simulink model "tasks100Hz"  (R2014a)
settings: Solver=FixedStepDiscrete  StartTime=0.0  StopTime=simTime  FixedStep=filterDT  RelTol=1e-3
values from neighbouring files (symbols this model uses):
  earthAccelDenHP = p    [setup.m]
  earthAccelNumHP = p    [setup.m]
  eepromConfig = p    [setup.m]
  filterDT = 1 / 100    (= 0.01)    [setup.m]
undefined symbols (not defined in the file or in its folder): DiscIntNeverNeededParam
libraries: simulink x7, aerolibutil x4, aerolibtransform2 x1
settings Model: Creator=John Ihlein  LastModifiedBy=John Ihlein
settings DataIOCC: SaveFormat=Structure  SaveOutput=off  SaveTime=off
settings OptimizationCC: InlineParams=on  DefaultUnderspecifiedDataType=single  InlineInvariantSignals=on  PassReuseOutputArgsAs=Individual arguments  StateBitsets=on  DataBitsets=on  ZeroExternalMemoryAtStartup=off  ZeroInternalMemoryAtStartup=off  EfficientFloat2IntCast=on  OptimizeModelRefInitCode=on  LifeSpan=1
settings DebuggingCC: ParameterPrecisionLossMsg=none  UniqueDataStoreMsg=error  AssertControl=DisableAll
settings HardwareCC: ProdLargestAtomicInteger=Integer  ProdLargestAtomicFloat=Float  ProdIntDivRoundTo=Zero  ProdEndianess=LittleEndian  ProdHWDeviceType=STMicroelectronics->STM32F4xx 32-bit Cortex-M4
settings RTWCC: SystemTargetFile=ert.tlc  GenCodeOnly=on  TemplateMakefile=ert_default_tmf  Description=Embedded Coder  ProcessScript=ert_make_rtw_hook
settings CodeAppCC: IgnoreCustomStorageClasses=off  IgnoreTestpoints=on
settings ERTTargetCC: ParMdlRefBuildCompliant=on  CompOptLevelCompliant=on  ConcurrentExecutionCompliant=on  IncludeMdlTerminateFcn=off  ERTFirstTimeCompliant=on  SupportNonFinite=off  ParenthesesLevel=Maximum  ModelStepFunctionPrototypeControlCompliant=on  CPPClassGenCompliant=on  InlinedParameterPlacement=Hierarchical  ERTCustomFileTemplate=example_file_process.tlc  ERTFilePackagingFormat=Compact

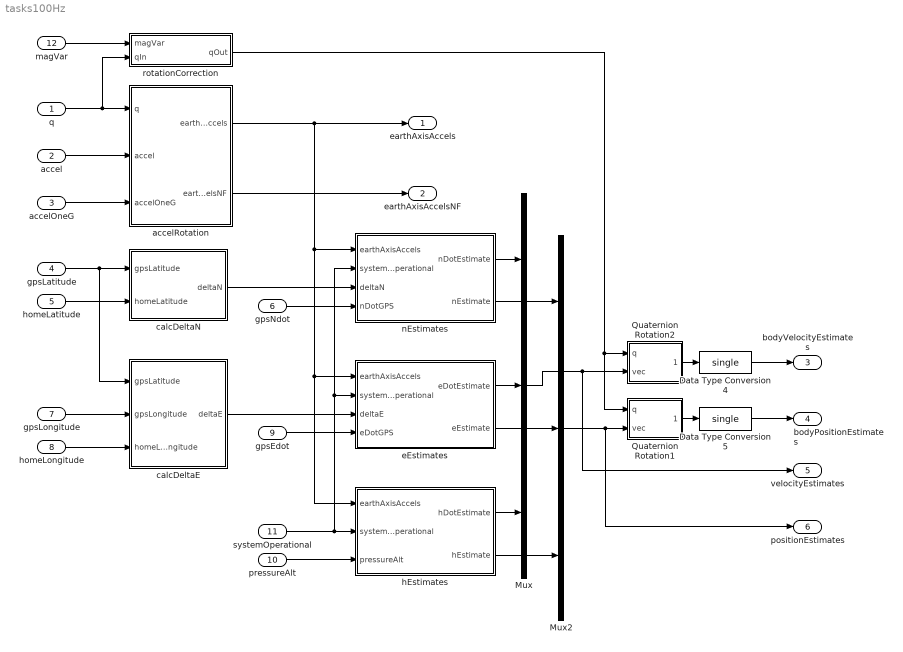
== system tasks100Hz ==
  q : Inport  OutDataTypeStr=single  PortDimensions=4  SampleTime=filterDT
  accel : Inport  Port=2  OutDataTypeStr=single  PortDimensions=3  SampleTime=filterDT
  accelOneG : Inport  Port=3  OutDataTypeStr=single  PortDimensions=1  SampleTime=filterDT
  gpsLatitude : Inport  Port=4  OutDataTypeStr=int32  PortDimensions=1  SampleTime=filterDT
  homeLatitude : Inport  Port=5  OutDataTypeStr=int32  PortDimensions=1  SampleTime=filterDT
  gpsNdot : Inport  Port=6  OutDataTypeStr=int32  PortDimensions=1  SampleTime=filterDT
  gpsLongitude : Inport  Port=7  OutDataTypeStr=int32  PortDimensions=1  SampleTime=filterDT
  homeLongitude : Inport  Port=8  OutDataTypeStr=int32  PortDimensions=1  SampleTime=filterDT
  gpsEdot : Inport  Port=9  OutDataTypeStr=int32  PortDimensions=1  SampleTime=filterDT
  pressureAlt : Inport  Port=10  OutDataTypeStr=single  PortDimensions=1  SampleTime=filterDT
  systemOperational : Inport  Port=11  OutDataTypeStr=uint8  PortDimensions=1  SampleTime=filterDT
  magVar : Inport  Port=12  OutDataTypeStr=single  PortDimensions=1  SampleTime=filterDT
  Data Type Conversion4 : DataTypeConversion  OutDataTypeStr=single
  Data Type Conversion5 : DataTypeConversion  OutDataTypeStr=single
  Mux : Mux  Inputs=3
  Mux2 : Mux  Inputs=3
  Quaternion Rotation1 : Subsystem
  Quaternion Rotation2 : Subsystem
  accelRotation : Subsystem  TreatAsAtomicUnit=on
  calcDeltaE : Subsystem  TreatAsAtomicUnit=on
  calcDeltaN : Subsystem  TreatAsAtomicUnit=on
  eEstimates : Subsystem  TreatAsAtomicUnit=on
  hEstimates : Subsystem  TreatAsAtomicUnit=on
  nEstimates : Subsystem  TreatAsAtomicUnit=on
  rotationCorrection : Subsystem  TreatAsAtomicUnit=on
  earthAxisAccels : Outport  OutDataTypeStr=single  PortDimensions=3  SampleTime=filterDT
  earthAxisAccelsNF : Outport  Port=2  OutDataTypeStr=single  PortDimensions=3  SampleTime=filterDT
  bodyVelocityEstimates : Outport  Port=3  OutDataTypeStr=single  PortDimensions=3  SampleTime=filterDT
  bodyPositionEstimates : Outport  Port=4  OutDataTypeStr=single  PortDimensions=3  SampleTime=filterDT
  velocityEstimates : Outport  Port=5  OutDataTypeStr=single  PortDimensions=3  SampleTime=filterDT
  positionEstimates : Outport  Port=6  OutDataTypeStr=single  PortDimensions=3  SampleTime=filterDT
  wires:
  systemOperational/1 -> nEstimates/2(systemOperational), eEstimates/2(systemOperational), hEstimates/2(systemOperational)
  pressureAlt/1 -> hEstimates/3(pressureAlt)
  hEstimates/1(hDotEstimate) -> Mux/3
  gpsNdot/1 -> nEstimates/4(nDotGPS)
  gpsEdot/1 -> eEstimates/4(eDotGPS)
  nEstimates/1(nDotEstimate) -> Mux/1
  nEstimates/2(nEstimate) -> Mux2/1
  eEstimates/1(eDotEstimate) -> Mux/2
  eEstimates/2(eEstimate) -> Mux2/2
  Quaternion Rotation2/1(vec_rot) -> Data Type Conversion4/1
  Quaternion Rotation1/1(vec_rot) -> Data Type Conversion5/1
  Data Type Conversion4/1 -> bodyVelocityEstimates/1
  Data Type Conversion5/1 -> bodyPositionEstimates/1
  hEstimates/2(hEstimate) -> Mux2/3
  Mux2/1 -> positionEstimates/1, Quaternion Rotation1/2(vec)
  accelOneG/1 -> accelRotation/3(accelOneG)
  homeLatitude/1 -> calcDeltaN/2(homeLatitude)
  calcDeltaN/1(deltaN) -> nEstimates/3(deltaN)
  gpsLongitude/1 -> calcDeltaE/2(gpsLongitude)
  homeLongitude/1 -> calcDeltaE/3(homeLongitude)
  calcDeltaE/1(deltaE) -> eEstimates/3(deltaE)
  gpsLatitude/1 -> calcDeltaN/1(gpsLatitude), calcDeltaE/1(gpsLatitude)
  q/1 -> rotationCorrection/2(qIn), accelRotation/1(q)
  accelRotation/2(earthAxisAccelsNF) -> earthAxisAccelsNF/1
  accelRotation/1(earthAxisAccels) -> eEstimates/1(earthAxisAccels), hEstimates/1(earthAxisAccels), nEstimates/1(earthAxisAccels), earthAxisAccels/1
  accel/1 -> accelRotation/2(accel)
  Mux/1 -> velocityEstimates/1, Quaternion Rotation2/2(vec)
  magVar/1 -> rotationCorrection/1(magVar)
  rotationCorrection/1(qOut) -> Quaternion Rotation2/1(q), Quaternion Rotation1/1(q)

== system tasks100Hz/Quaternion Rotation1 ==
  q : Inport
  vec : Inport  Port=2
  Mux1 : Mux  Inputs=3
  Quaternion Normalize : aerolibutil/Quaternion Normalize
  singleV1 : Subsystem
  singleV2 : Subsystem
  singleV3 : Subsystem
  vec_rot : Outport
  wires:
  q/1 -> Quaternion Normalize/1
  singleV1/1(V1) -> Mux1/1
  vec/1 -> singleV1/2(vec), singleV3/2(vec), singleV2/2(vec)
  Quaternion Normalize/1 -> singleV1/1(q), singleV3/1(q), singleV2/1(q)
  Mux1/1 -> vec_rot/1
  singleV3/1(V3) -> Mux1/3
  singleV2/1(V2) -> Mux1/2

== system tasks100Hz/Quaternion Rotation2 ==
  q : Inport
  vec : Inport  Port=2
  Mux1 : Mux  Inputs=3
  Quaternion Normalize : aerolibutil/Quaternion Normalize
  singleV1 : Subsystem
  singleV2 : Subsystem
  singleV3 : Subsystem
  vec_rot : Outport
  wires:
  singleV2/1(V2) -> Mux1/2
  singleV3/1(V3) -> Mux1/3
  Mux1/1 -> vec_rot/1
  Quaternion Normalize/1 -> singleV2/1(q), singleV3/1(q), singleV1/1(q)
  vec/1 -> singleV2/2(vec), singleV3/2(vec), singleV1/2(vec)
  singleV1/1(V1) -> Mux1/1
  q/1 -> Quaternion Normalize/1

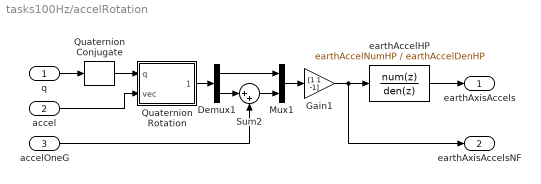
== system tasks100Hz/accelRotation ==
  q : Inport
  accel : Inport  Port=2
  accelOneG : Inport  Port=3
  Demux1 : Demux  Outputs=[2 1]
  Gain1 : Gain  Gain=[1 1 -1]
  Mux1 : Mux  Inputs=[2 1]
  Quaternion Conjugate : aerolibutil/Quaternion Conjugate
  Quaternion Rotation : Subsystem
  Sum2 : Sum  Inputs=|++
  earthAccelHP : DiscreteTransferFcn  Numerator=earthAccelNumHP  Denominator=earthAccelDenHP
  earthAxisAccels : Outport
  earthAxisAccelsNF : Outport  Port=2
  wires:
  Gain1/1 -> earthAxisAccelsNF/1, earthAccelHP/1
  accelOneG/1 -> Sum2/2
  Demux1/1 -> Mux1/1
  Sum2/1 -> Mux1/2
  Demux1/2 -> Sum2/1
  Quaternion Conjugate/1 -> Quaternion Rotation/1(q)
  accel/1 -> Quaternion Rotation/2(vec)
  q/1 -> Quaternion Conjugate/1
  Quaternion Rotation/1(vec_rot) -> Demux1/1
  Mux1/1 -> Gain1/1
  earthAccelHP/1 -> earthAxisAccels/1

== system tasks100Hz/calcDeltaE ==
  gpsLatitude : Inport
  gpsLongitude : Inport  Port=2
  homeLongitude : Inport  Port=3
  Data Type Conversion2 : DataTypeConversion  OutDataTypeStr=single
  Data Type Conversion3 : DataTypeConversion  OutDataTypeStr=single
  Gain1 : Gain  Gain=pi / 180 * 1e-7
  Gain2 : Gain  Gain=0.01111949
  Product : Product
  Sum2 : Sum  Inputs=|+-
  Trigonometric Function : Trigonometry  Operator=cos
  stdRadianLimit : Subsystem
  deltaE : Outport
  wires:
  stdRadianLimit/1(stdDegrees) -> Gain2/1
  gpsLatitude/1 -> Data Type Conversion2/1
  Data Type Conversion3/1 -> stdRadianLimit/1(degrees)
  Product/1 -> deltaE/1
  Sum2/1 -> Data Type Conversion3/1
  homeLongitude/1 -> Sum2/2
  Gain2/1 -> Product/2
  Trigonometric Function/1 -> Product/1
  Gain1/1 -> Trigonometric Function/1
  Data Type Conversion2/1 -> Gain1/1
  gpsLongitude/1 -> Sum2/1

== system tasks100Hz/calcDeltaN ==
  gpsLatitude : Inport
  homeLatitude : Inport  Port=2
  Data Type Conversion1 : DataTypeConversion  OutDataTypeStr=single
  Gain : Gain  Gain=0.01111949
  Sum1 : Sum  Inputs=|+-
  deltaN : Outport
  wires:
  Sum1/1 -> Data Type Conversion1/1
  homeLatitude/1 -> Sum1/2
  Data Type Conversion1/1 -> Gain/1
  gpsLatitude/1 -> Sum1/1
  Gain/1 -> deltaN/1

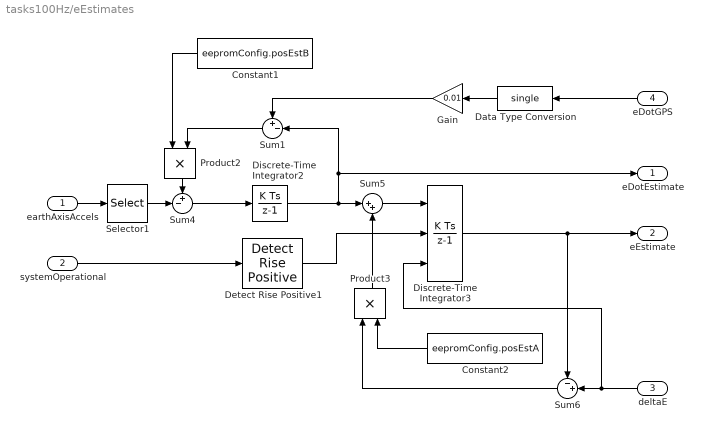
== system tasks100Hz/eEstimates ==
  earthAxisAccels : Inport
  systemOperational : Inport  Port=2
  deltaE : Inport  Port=3
  eDotGPS : Inport  Port=4  OutDataTypeStr=int32
  Constant1 : Constant  Value=eepromConfig.posEstB  SampleTime=filterDT
  Constant2 : Constant  Value=eepromConfig.posEstA  SampleTime=filterDT
  Data Type Conversion : DataTypeConversion  OutDataTypeStr=single
  Detect Rise Positive1 : simulink/Logic and Bit Operations/Detect Rise Positive  vinit=0  InputProcessing=Inherited  OutDataTypeStr=boolean
  Discrete-Time Integrator2 : DiscreteIntegrator  SampleTime=filterDT  ICPrevOutput=DiscIntNeverNeededParam  ICPrevScaledInput=DiscIntNeverNeededParam
  Discrete-Time Integrator3 : DiscreteIntegrator  ExternalReset=rising  InitialConditionSource=external  SampleTime=filterDT  ICPrevOutput=DiscIntNeverNeededParam  ICPrevScaledInput=DiscIntNeverNeededParam
  Gain : Gain  Gain=0.01
  Product2 : Product
  Product3 : Product
  Selector1 : Selector  IndexMode=Zero-based  InputPortWidth=3
  Sum1 : Sum  Inputs=+-|
  Sum4 : Sum  Inputs=+-|
  Sum5 : Sum  Inputs=|++
  Sum6 : Sum  Inputs=-+|
  eDotEstimate : Outport
  eEstimate : Outport  Port=2
  wires:
  Data Type Conversion/1 -> Gain/1
  Gain/1 -> Sum1/1
  eDotGPS/1 -> Data Type Conversion/1
  Sum1/1 -> Product2/2
  Constant1/1 -> Product2/1
  Product2/1 -> Sum4/1
  Selector1/1 -> Sum4/2
  Sum4/1 -> Discrete-Time Integrator2/1
  Product3/1 -> Sum5/2
  Detect Rise Positive1/1 -> Discrete-Time Integrator3/2
  Constant2/1 -> Product3/2
  Discrete-Time Integrator3/1 -> eEstimate/1, Sum6/1
  Sum6/1 -> Product3/1
  Discrete-Time Integrator2/1 -> eDotEstimate/1, Sum1/2, Sum5/1
  Sum5/1 -> Discrete-Time Integrator3/1
  earthAxisAccels/1 -> Selector1/1
  deltaE/1 -> Discrete-Time Integrator3/3, Sum6/2
  systemOperational/1 -> Detect Rise Positive1/1

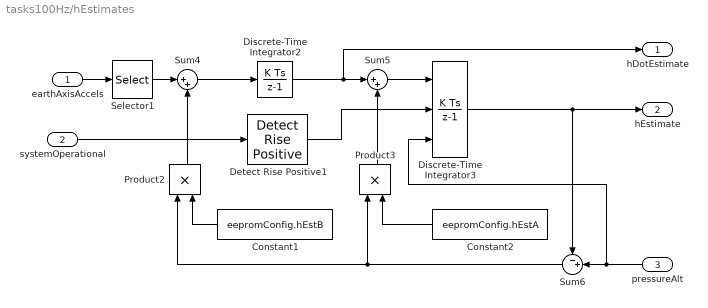
== system tasks100Hz/hEstimates ==
  earthAxisAccels : Inport
  systemOperational : Inport  Port=2
  pressureAlt : Inport  Port=3
  Constant1 : Constant  Value=eepromConfig.hEstB  SampleTime=filterDT
  Constant2 : Constant  Value=eepromConfig.hEstA  SampleTime=filterDT
  Detect Rise Positive1 : simulink/Logic and Bit Operations/Detect Rise Positive  vinit=0  InputProcessing=Inherited  OutDataTypeStr=boolean
  Discrete-Time Integrator2 : DiscreteIntegrator  SampleTime=filterDT  ICPrevOutput=DiscIntNeverNeededParam  ICPrevScaledInput=DiscIntNeverNeededParam
  Discrete-Time Integrator3 : DiscreteIntegrator  ExternalReset=rising  InitialConditionSource=external  SampleTime=filterDT  ICPrevOutput=DiscIntNeverNeededParam  ICPrevScaledInput=DiscIntNeverNeededParam
  Product2 : Product
  Product3 : Product
  Selector1 : Selector  IndexMode=Zero-based  InputPortWidth=3  Indices=2
  Sum4 : Sum  Inputs=|++
  Sum5 : Sum  Inputs=|++
  Sum6 : Sum  Inputs=-+|
  hDotEstimate : Outport
  hEstimate : Outport  Port=2
  wires:
  systemOperational/1 -> Detect Rise Positive1/1
  pressureAlt/1 -> Sum6/2, Discrete-Time Integrator3/3
  earthAxisAccels/1 -> Selector1/1
  Sum5/1 -> Discrete-Time Integrator3/1
  Discrete-Time Integrator2/1 -> Sum5/1, hDotEstimate/1
  Sum6/1 -> Product3/1, Product2/1
  Discrete-Time Integrator3/1 -> Sum6/1, hEstimate/1
  Constant2/1 -> Product3/2
  Selector1/1 -> Sum4/1
  Detect Rise Positive1/1 -> Discrete-Time Integrator3/2
  Product3/1 -> Sum5/2
  Sum4/1 -> Discrete-Time Integrator2/1
  Constant1/1 -> Product2/2
  Product2/1 -> Sum4/2

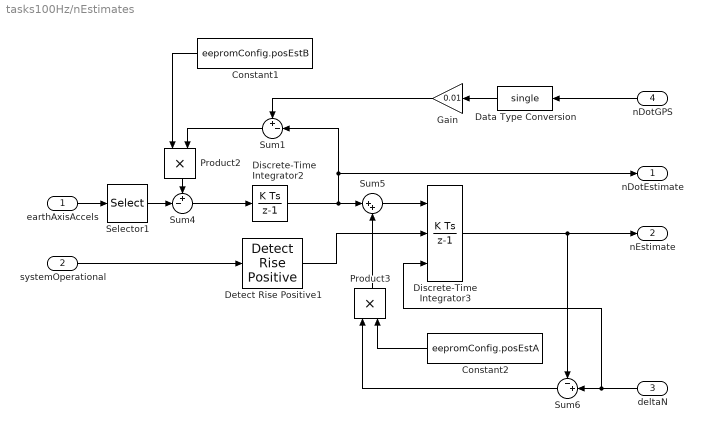
== system tasks100Hz/nEstimates ==
  earthAxisAccels : Inport
  systemOperational : Inport  Port=2
  deltaN : Inport  Port=3
  nDotGPS : Inport  Port=4  OutDataTypeStr=int32
  Constant1 : Constant  Value=eepromConfig.posEstB  SampleTime=filterDT
  Constant2 : Constant  Value=eepromConfig.posEstA  SampleTime=filterDT
  Data Type Conversion : DataTypeConversion  OutDataTypeStr=single
  Detect Rise Positive1 : simulink/Logic and Bit Operations/Detect Rise Positive  vinit=0  InputProcessing=Inherited  OutDataTypeStr=boolean
  Discrete-Time Integrator2 : DiscreteIntegrator  SampleTime=filterDT  ICPrevOutput=DiscIntNeverNeededParam  ICPrevScaledInput=DiscIntNeverNeededParam
  Discrete-Time Integrator3 : DiscreteIntegrator  ExternalReset=rising  InitialConditionSource=external  SampleTime=filterDT  ICPrevOutput=DiscIntNeverNeededParam  ICPrevScaledInput=DiscIntNeverNeededParam
  Gain : Gain  Gain=0.01
  Product2 : Product
  Product3 : Product
  Selector1 : Selector  IndexMode=Zero-based  InputPortWidth=3  Indices=0
  Sum1 : Sum  Inputs=+-|
  Sum4 : Sum  Inputs=+-|
  Sum5 : Sum  Inputs=|++
  Sum6 : Sum  Inputs=-+|
  nDotEstimate : Outport
  nEstimate : Outport  Port=2
  wires:
  systemOperational/1 -> Detect Rise Positive1/1
  deltaN/1 -> Sum6/2, Discrete-Time Integrator3/3
  earthAxisAccels/1 -> Selector1/1
  Sum5/1 -> Discrete-Time Integrator3/1
  Discrete-Time Integrator2/1 -> Sum5/1, Sum1/2, nDotEstimate/1
  Sum6/1 -> Product3/1
  Discrete-Time Integrator3/1 -> Sum6/1, nEstimate/1
  Constant2/1 -> Product3/2
  Detect Rise Positive1/1 -> Discrete-Time Integrator3/2
  Product3/1 -> Sum5/2
  Sum4/1 -> Discrete-Time Integrator2/1
  Selector1/1 -> Sum4/2
  Product2/1 -> Sum4/1
  Constant1/1 -> Product2/1
  Sum1/1 -> Product2/2
  nDotGPS/1 -> Data Type Conversion/1
  Gain/1 -> Sum1/1
  Data Type Conversion/1 -> Gain/1

== system tasks100Hz/rotationCorrection ==
  magVar : Inport
  qIn : Inport  Port=2
  Demux : Demux  Outputs=[1 2]
  Gain3 : Gain  Gain=[1 0 0]
  Mux : Mux  Inputs=[1 2]
  Quaternions to Rotation Angles : aerolibtransform2/Quaternions to Rotation Angles  rotationOrder=ZYX
  Rotation Angles to Quaternions Rotation Order: ZYX : Subsystem
  Sum : Sum  Inputs=++|
  stdRadianLimit : Subsystem
  qOut : Outport
  wires:
  Mux/1 -> Rotation Angles to Quaternions Rotation Order: ZYX/1("R1, R2, R3")
  Gain3/1 -> Demux/1
  stdRadianLimit/1(stdRadians) -> Mux/1
  Demux/1 -> Sum/2
  Demux/2 -> Mux/2
  magVar/1 -> Sum/1
  Sum/1 -> stdRadianLimit/1(radians)
  qIn/1 -> Quaternions to Rotation Angles/1
  Quaternions to Rotation Angles/1 -> Gain3/1
  Rotation Angles to Quaternions Rotation Order: ZYX/1(q) -> qOut/1

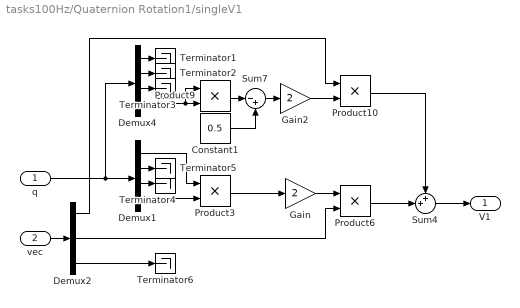
== system tasks100Hz/Quaternion Rotation1/singleV1 ==
  q : Inport
  vec : Inport  Port=2
  Constant1 : Constant  Value=0.5  OutDataTypeStr=single
  Demux1 : Demux
  Demux2 : Demux  Outputs=3
  Demux4 : Demux
  Gain : Gain  Gain=2
  Gain2 : Gain  Gain=2
  Product{3,6,9..10} (4 alike) : Product  RndMeth=Zero
  Sum4 : Sum  Inputs=++|
  Sum7 : Sum  Inputs=|-+
  Terminator{1..6} (6 alike) : Terminator
  V1 : Outport
  wires:
  Product6/1 -> Sum4/2
  Sum4/1 -> V1/1
  q/1 -> Demux4/1, Demux1/1
  vec/1 -> Demux2/1
  Demux1/4 -> Product3/2
  Demux1/1 -> Product3/1
  Product3/1 -> Gain/1
  Product10/1 -> Sum4/1
  Demux4/2 -> Terminator2/1
  Gain/1 -> Product6/1
  Gain2/1 -> Product10/2
  Demux2/2 -> Product6/2
  Demux2/1 -> Product10/1
  Sum7/1 -> Gain2/1
  Demux4/1 -> Terminator1/1
  Demux4/3 -> Terminator3/1
  Demux4/4 -> Product9/1, Product9/2
  Product9/1 -> Sum7/1
  Constant1/1 -> Sum7/2
  Demux1/3 -> Terminator4/1
  Demux1/2 -> Terminator5/1
  Demux2/3 -> Terminator6/1

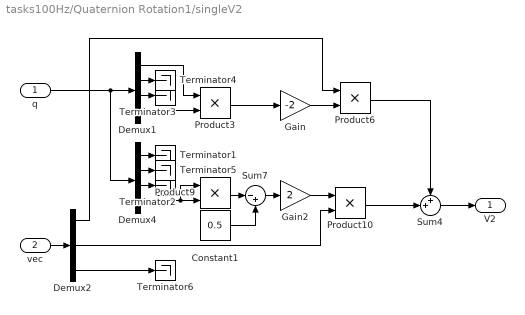
== system tasks100Hz/Quaternion Rotation1/singleV2 ==
  q : Inport
  vec : Inport  Port=2
  Constant1 : Constant  Value=0.5  OutDataTypeStr=single
  Demux1 : Demux
  Demux2 : Demux  Outputs=3
  Demux4 : Demux
  Gain : Gain  Gain=-2
  Gain2 : Gain  Gain=2
  Product{3,6,9..10} (4 alike) : Product  RndMeth=Zero
  Sum4 : Sum  Inputs=++|
  Sum7 : Sum  Inputs=|-+
  Terminator{1..6} (6 alike) : Terminator
  V2 : Outport
  wires:
  Demux1/1 -> Product3/1
  Demux1/4 -> Product3/2
  Gain/1 -> Product6/2
  Sum7/1 -> Gain2/1
  Product10/1 -> Sum4/2
  Demux4/1 -> Terminator1/1
  Sum4/1 -> V2/1
  Demux4/4 -> Product9/1, Product9/2
  q/1 -> Demux1/1, Demux4/1
  vec/1 -> Demux2/1
  Demux2/1 -> Product6/1
  Demux2/2 -> Product10/2
  Demux4/3 -> Terminator2/1
  Gain2/1 -> Product10/1
  Product6/1 -> Sum4/1
  Product3/1 -> Gain/1
  Demux1/2 -> Terminator4/1
  Demux1/3 -> Terminator3/1
  Constant1/1 -> Sum7/2
  Product9/1 -> Sum7/1
  Demux4/2 -> Terminator5/1
  Demux2/3 -> Terminator6/1

== system tasks100Hz/Quaternion Rotation1/singleV3 ==
  q : Inport
  vec : Inport  Port=2
  Demux2 : Demux  Outputs=3
  Terminator1 : Terminator
  Terminator2 : Terminator
  Terminator3 : Terminator
  V3 : Outport
  wires:
  vec/1 -> Demux2/1
  Demux2/1 -> Terminator2/1
  Demux2/2 -> Terminator3/1
  Demux2/3 -> V3/1
  q/1 -> Terminator1/1

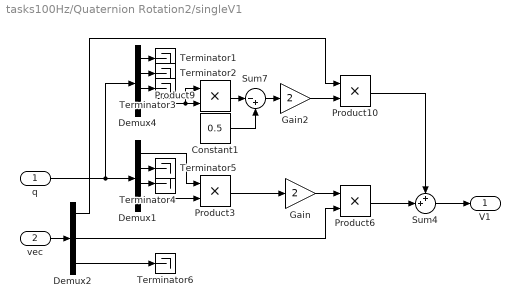
== system tasks100Hz/Quaternion Rotation2/singleV1 ==
  q : Inport
  vec : Inport  Port=2
  Constant1 : Constant  Value=0.5  OutDataTypeStr=single
  Demux1 : Demux
  Demux2 : Demux  Outputs=3
  Demux4 : Demux
  Gain : Gain  Gain=2
  Gain2 : Gain  Gain=2
  Product{3,6,9..10} (4 alike) : Product  RndMeth=Zero
  Sum4 : Sum  Inputs=++|
  Sum7 : Sum  Inputs=|-+
  Terminator{1..6} (6 alike) : Terminator
  V1 : Outport
  wires:
  Demux2/3 -> Terminator6/1
  Demux1/2 -> Terminator5/1
  Demux1/3 -> Terminator4/1
  Constant1/1 -> Sum7/2
  Product9/1 -> Sum7/1
  Demux4/4 -> Product9/2, Product9/1
  Demux4/3 -> Terminator3/1
  Demux4/1 -> Terminator1/1
  Sum7/1 -> Gain2/1
  Demux2/1 -> Product10/1
  Demux2/2 -> Product6/2
  Gain2/1 -> Product10/2
  Gain/1 -> Product6/1
  Demux4/2 -> Terminator2/1
  Product10/1 -> Sum4/1
  Product3/1 -> Gain/1
  Demux1/1 -> Product3/1
  Demux1/4 -> Product3/2
  vec/1 -> Demux2/1
  q/1 -> Demux1/1, Demux4/1
  Sum4/1 -> V1/1
  Product6/1 -> Sum4/2

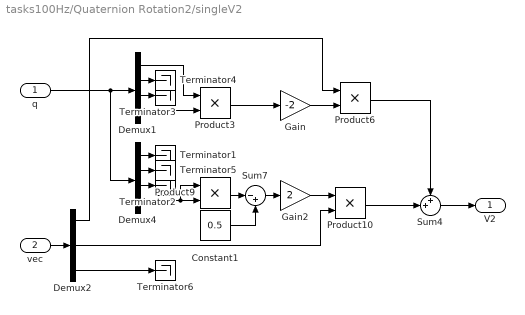
== system tasks100Hz/Quaternion Rotation2/singleV2 ==
  q : Inport
  vec : Inport  Port=2
  Constant1 : Constant  Value=0.5  OutDataTypeStr=single
  Demux1 : Demux
  Demux2 : Demux  Outputs=3
  Demux4 : Demux
  Gain : Gain  Gain=-2
  Gain2 : Gain  Gain=2
  Product{3,6,9..10} (4 alike) : Product  RndMeth=Zero
  Sum4 : Sum  Inputs=++|
  Sum7 : Sum  Inputs=|-+
  Terminator{1..6} (6 alike) : Terminator
  V2 : Outport
  wires:
  Demux2/3 -> Terminator6/1
  Demux4/2 -> Terminator5/1
  Product9/1 -> Sum7/1
  Constant1/1 -> Sum7/2
  Demux1/3 -> Terminator3/1
  Demux1/2 -> Terminator4/1
  Product3/1 -> Gain/1
  Product6/1 -> Sum4/1
  Gain2/1 -> Product10/1
  Demux4/3 -> Terminator2/1
  Demux2/2 -> Product10/2
  Demux2/1 -> Product6/1
  vec/1 -> Demux2/1
  q/1 -> Demux4/1, Demux1/1
  Demux4/4 -> Product9/2, Product9/1
  Sum4/1 -> V2/1
  Demux4/1 -> Terminator1/1
  Product10/1 -> Sum4/2
  Sum7/1 -> Gain2/1
  Gain/1 -> Product6/2
  Demux1/4 -> Product3/2
  Demux1/1 -> Product3/1

== system tasks100Hz/Quaternion Rotation2/singleV3 ==
  q : Inport
  vec : Inport  Port=2
  Demux2 : Demux  Outputs=3
  Terminator1 : Terminator
  Terminator2 : Terminator
  Terminator3 : Terminator
  V3 : Outport
  wires:
  q/1 -> Terminator1/1
  Demux2/3 -> V3/1
  Demux2/2 -> Terminator3/1
  Demux2/1 -> Terminator2/1
  vec/1 -> Demux2/1

== system tasks100Hz/accelRotation/Quaternion Rotation ==
  q : Inport
  vec : Inport  Port=2
  Mux1 : Mux  Inputs=3
  Quaternion Normalize : aerolibutil/Quaternion Normalize
  singleV1 : Subsystem
  singleV2 : Subsystem
  singleV3 : Subsystem
  vec_rot : Outport
  wires:
  singleV2/1(V2) -> Mux1/2
  singleV3/1(V3) -> Mux1/3
  Mux1/1 -> vec_rot/1
  Quaternion Normalize/1 -> singleV2/1(q), singleV3/1(q), singleV1/1(q)
  vec/1 -> singleV2/2(vec), singleV3/2(vec), singleV1/2(vec)
  singleV1/1(V1) -> Mux1/1
  q/1 -> Quaternion Normalize/1

== system tasks100Hz/calcDeltaE/stdRadianLimit ==
  degrees : Inport
  Bias : Bias  Bias=- 360e7
  Bias1 : Bias  Bias=360e7
  Compare To Constant : simulink/Logic and Bit Operations/Compare To Constant  relop=>=  const=180e7  OutDataTypeStr=boolean
  Compare To Constant1 : simulink/Logic and Bit Operations/Compare To Constant  relop=<  const=-180e7  OutDataTypeStr=boolean
  Switch : Switch  Criteria=u2 > Threshold
  Switch1 : Switch  Criteria=u2 > Threshold
  stdDegrees : Outport
  wires:
  Switch/1 -> stdDegrees/1
  degrees/1 -> Bias/1, Compare To Constant/1, Bias1/1, Compare To Constant1/1, Switch1/3
  Switch1/1 -> Switch/3
  Compare To Constant1/1 -> Switch1/2
  Bias1/1 -> Switch1/1
  Bias/1 -> Switch/1
  Compare To Constant/1 -> Switch/2

== system tasks100Hz/rotationCorrection/Rotation Angles to Quaternions Rotation Order: ZYX ==
  "R1, R2, R3" : Inport
  1/2 : Gain  Gain=0.5  SaturateOnIntegerOverflow=on  OutDataTypeStr=Inherit: Same as input  ParamDataTypeStr=Inherit: Same as input
  Mux4 : Mux
  Selector : Selector  IndexMode=Zero-based  InputPortWidth=3  Indices=0
  Trigonometric Function : Trigonometry
  Trigonometric Function1 : Trigonometry  Operator=cos
  q1 : Constant  Value=0  OutDataTypeStr=single
  q2 : Constant  Value=0  OutDataTypeStr=single
  q : Outport
  wires:
  Selector/1 -> 1/2/1
  "R1, R2, R3"/1 -> Selector/1
  q1/1 -> Mux4/2
  Trigonometric Function1/1 -> Mux4/1
  1/2/1 -> Trigonometric Function/1, Trigonometric Function1/1
  q2/1 -> Mux4/3
  Trigonometric Function/1 -> Mux4/4
  Mux4/1 -> q/1

== system tasks100Hz/rotationCorrection/stdRadianLimit ==
  radians : Inport
  Bias : Bias  Bias=- 2*pi
  Bias1 : Bias  Bias=2*pi
  Compare To Constant : simulink/Logic and Bit Operations/Compare To Constant  relop=>=  const=pi  OutDataTypeStr=boolean
  Compare To Constant1 : simulink/Logic and Bit Operations/Compare To Constant  relop=<  const=-pi  OutDataTypeStr=boolean
  Switch : Switch  Criteria=u2 > Threshold
  Switch1 : Switch  Criteria=u2 > Threshold
  stdRadians : Outport
  wires:
  Switch/1 -> stdRadians/1
  radians/1 -> Bias/1, Compare To Constant/1, Bias1/1, Compare To Constant1/1, Switch1/3
  Switch1/1 -> Switch/3
  Compare To Constant1/1 -> Switch1/2
  Bias1/1 -> Switch1/1
  Bias/1 -> Switch/1
  Compare To Constant/1 -> Switch/2

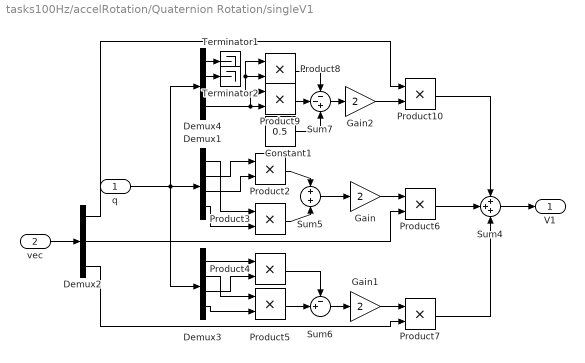
== system tasks100Hz/accelRotation/Quaternion Rotation/singleV1 ==
  q : Inport
  vec : Inport  Port=2
  Constant1 : Constant  Value=0.5  OutDataTypeStr=single
  Demux1 : Demux
  Demux2 : Demux  Outputs=3
  Demux3 : Demux
  Demux4 : Demux
  Gain : Gain  Gain=2
  Gain1 : Gain  Gain=2
  Gain2 : Gain  Gain=2
  Product{2..10} (9 alike) : Product  RndMeth=Zero
  Sum4 : Sum  Inputs=3
  Sum5 : Sum  Inputs=+|+
  Sum6 : Sum  Inputs=-+|
  Sum7 : Sum  Inputs=--+
  Terminator1 : Terminator
  Terminator2 : Terminator
  V1 : Outport
  wires:
  Demux4/3 -> Product8/2, Product8/1
  Demux4/4 -> Product9/1, Product9/2
  Demux4/1 -> Terminator1/1
  Sum7/1 -> Gain2/1
  Product4/1 -> Sum6/1
  Constant1/1 -> Sum7/3
  Demux2/1 -> Product10/1
  Sum6/1 -> Gain1/1
  Demux2/2 -> Product6/2
  Demux3/1 -> Product4/1
  Product5/1 -> Sum6/2
  Gain2/1 -> Product10/2
  Demux3/3 -> Product4/2
  Demux3/4 -> Product5/2
  Product8/1 -> Sum7/1
  Product9/1 -> Sum7/2
  Demux1/2 -> Product2/1
  Gain/1 -> Product6/1
  Demux4/2 -> Terminator2/1
  Product10/1 -> Sum4/1
  Demux3/2 -> Product5/1
  Demux2/3 -> Product7/2
  Product7/1 -> Sum4/3
  Sum5/1 -> Gain/1
  Demux1/1 -> Product3/1
  Demux1/4 -> Product3/2
  Demux1/3 -> Product2/2
  vec/1 -> Demux2/1
  q/1 -> Demux1/1, Demux4/1, Demux3/1
  Sum4/1 -> V1/1
  Product2/1 -> Sum5/1
  Product6/1 -> Sum4/2
  Product3/1 -> Sum5/2
  Gain1/1 -> Product7/1

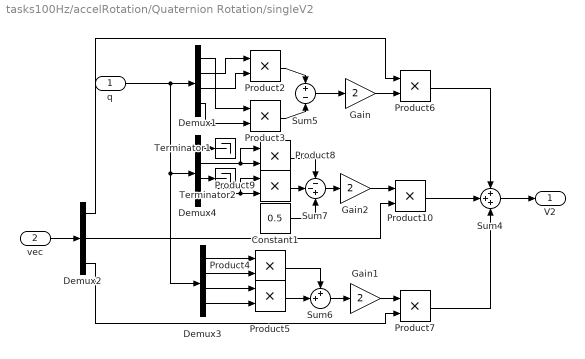
== system tasks100Hz/accelRotation/Quaternion Rotation/singleV2 ==
  q : Inport
  vec : Inport  Port=2
  Constant1 : Constant  Value=0.5  OutDataTypeStr=single
  Demux1 : Demux
  Demux2 : Demux  Outputs=3
  Demux3 : Demux
  Demux4 : Demux
  Gain : Gain  Gain=2
  Gain1 : Gain  Gain=2
  Gain2 : Gain  Gain=2
  Product{2..10} (9 alike) : Product  RndMeth=Zero
  Sum4 : Sum  Inputs=3
  Sum5 : Sum  Inputs=+|-
  Sum6 : Sum  Inputs=++|
  Sum7 : Sum  Inputs=--+
  Terminator1 : Terminator
  Terminator2 : Terminator
  V2 : Outport
  wires:
  Product9/1 -> Sum7/2
  Product6/1 -> Sum4/1
  Gain2/1 -> Product10/1
  Product4/1 -> Sum6/1
  Demux4/3 -> Terminator2/1
  Demux2/2 -> Product10/2
  Demux2/1 -> Product6/1
  Demux2/3 -> Product7/2
  Product3/1 -> Sum5/2
  Product2/1 -> Sum5/1
  vec/1 -> Demux2/1
  q/1 -> Demux4/1, Demux3/1, Demux1/1
  Demux1/2 -> Product2/1
  Gain1/1 -> Product7/1
  Demux3/2 -> Product4/2
  Demux3/3 -> Product5/1
  Demux3/4 -> Product5/2
  Demux4/4 -> Product9/2, Product9/1
  Sum6/1 -> Gain1/1
  Demux3/1 -> Product4/1
  Sum4/1 -> V2/1
  Demux4/1 -> Terminator1/1
  Product7/1 -> Sum4/3
  Product8/1 -> Sum7/1
  Constant1/1 -> Sum7/3
  Product10/1 -> Sum4/2
  Demux1/3 -> Product2/2
  Demux4/2 -> Product8/1, Product8/2
  Product5/1 -> Sum6/2
  Sum7/1 -> Gain2/1
  Sum5/1 -> Gain/1
  Gain/1 -> Product6/2
  Demux1/4 -> Product3/2
  Demux1/1 -> Product3/1

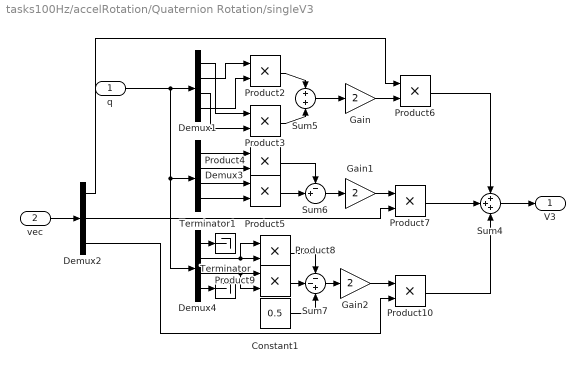
== system tasks100Hz/accelRotation/Quaternion Rotation/singleV3 ==
  q : Inport
  vec : Inport  Port=2
  Constant1 : Constant  Value=0.5  OutDataTypeStr=single
  Demux1 : Demux
  Demux2 : Demux  Outputs=3
  Demux3 : Demux
  Demux4 : Demux
  Gain : Gain  Gain=2
  Gain1 : Gain  Gain=2
  Gain2 : Gain  Gain=2
  Product{2..10} (9 alike) : Product  RndMeth=Zero
  Sum4 : Sum  Inputs=3
  Sum5 : Sum  Inputs=+|+
  Sum6 : Sum  Inputs=-+|
  Sum7 : Sum  Inputs=--+
  Terminator : Terminator
  Terminator1 : Terminator
  V3 : Outport
  wires:
  Demux2/3 -> Product10/2
  Constant1/1 -> Sum7/3
  Demux4/1 -> Terminator1/1
  Demux4/4 -> Terminator/1
  Gain2/1 -> Product10/1
  Sum7/1 -> Gain2/1
  Product9/1 -> Sum7/2
  Product8/1 -> Sum7/1
  Demux4/3 -> Product9/1, Product9/2
  Demux4/2 -> Product8/2, Product8/1
  Product6/1 -> Sum4/1
  Product7/1 -> Sum4/2
  Demux2/2 -> Product7/2
  Gain1/1 -> Product7/1
  Demux3/4 -> Product5/2
  Demux3/3 -> Product5/1
  Demux3/2 -> Product4/2
  Demux3/1 -> Product4/1
  Sum6/1 -> Gain1/1
  Product4/1 -> Sum6/1
  Product5/1 -> Sum6/2
  Demux2/1 -> Product6/1
  Gain/1 -> Product6/2
  Sum5/1 -> Gain/1
  Demux1/3 -> Product3/2
  Demux1/1 -> Product3/1
  Demux1/2 -> Product2/1
  Demux1/4 -> Product2/2
  q/1 -> Demux1/1, Demux3/1, Demux4/1
  vec/1 -> Demux2/1
  Product2/1 -> Sum5/1
  Product3/1 -> Sum5/2
  Sum4/1 -> V3/1
  Product10/1 -> Sum4/3
